simulink model "pathestimator"  (R2016a)
settings: Solver=VariableStepAuto  StartTime=0.0  StopTime=10.0  RelTol=1e-3
settings Model: Creator=s162602  LastModifiedBy=s162602

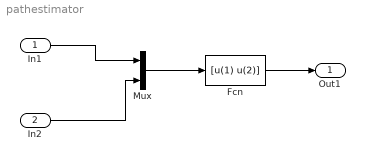
== system pathestimator ==
  In1 : Inport
  In2 : Inport  Port=2
  Fcn : Fcn  Expr=[u(1) u(2)]
  Mux : Mux  Inputs=2
  Out1 : Outport
  wires:
  In1/1 -> Mux/1
  In2/1 -> Mux/2
  Mux/1 -> Fcn/1
  Fcn/1 -> Out1/1
